simulink model "buck_converter_closed_loop_with_cascaded_comp"  (R2019a)
settings: Solver=VariableStepAuto  StartTime=0.0  StopTime=0.5  MaxStep=1e-6  RelTol=1e-6
values from neighbouring files (symbols this model uses):
  C = 68e-6    (= 6.8e-05)    [parameters_closed_loop_with_various_load.m]
  Cc2 = 2.8e-9    (= 2.8e-09)    [parameters_closed_loop_with_various_load.m]
  Cc3 = 470e-12    (= 4.7e-10)    [parameters_closed_loop_with_various_load.m]
  Cv2 = 0.94e-6    (= 9.4e-07)    [parameters_closed_loop_with_various_load.m]
  Cv3 = 0.056e-6    (= 5.6e-08)    [parameters_closed_loop_with_various_load.m]
  H = 0.5    [parameters_closed_loop_with_various_load.m]
  L = 68e-6    (= 6.8e-05)    [parameters_closed_loop_with_various_load.m]
  R = V/I    (= 0.363636363636)    [parameters_closed_loop_with_various_load.m]
  Ra = 2e3    (= 2000)    [parameters_closed_loop_with_various_load.m]
  Rb = 2e3    (= 2000)    [parameters_closed_loop_with_various_load.m]
  Rc1 = 1e3    (= 1000)    [parameters_closed_loop_with_various_load.m]
  Rc2 = 13.3404e3    (= 13340.4)    [parameters_closed_loop_with_various_load.m]
  Resr = 9e-3    (= 0.009)    [parameters_closed_loop_with_various_load.m]
  Rf = 0.3    [parameters_closed_loop_with_various_load.m]
  RL = 30e-3    (= 0.03)    [parameters_closed_loop_with_various_load.m]
  Rv2 = 546    [parameters_closed_loop_with_various_load.m]
  V = 1.2    [parameters_closed_loop_with_various_load.m]
  Vm = 5    [parameters_closed_loop_with_various_load.m]
undefined symbols (not defined in the file or in its folder): Rcomp_1
libraries: powerlib x64, simulink x1, powerlib_meascontrol x1
settings Model: Creator=Görkem  LastModifiedBy=Görkem
settings SolverCC: ZeroCrossAlgorithm=Adaptive
settings DebuggingCC: IgnoredZcDiagnostic=none

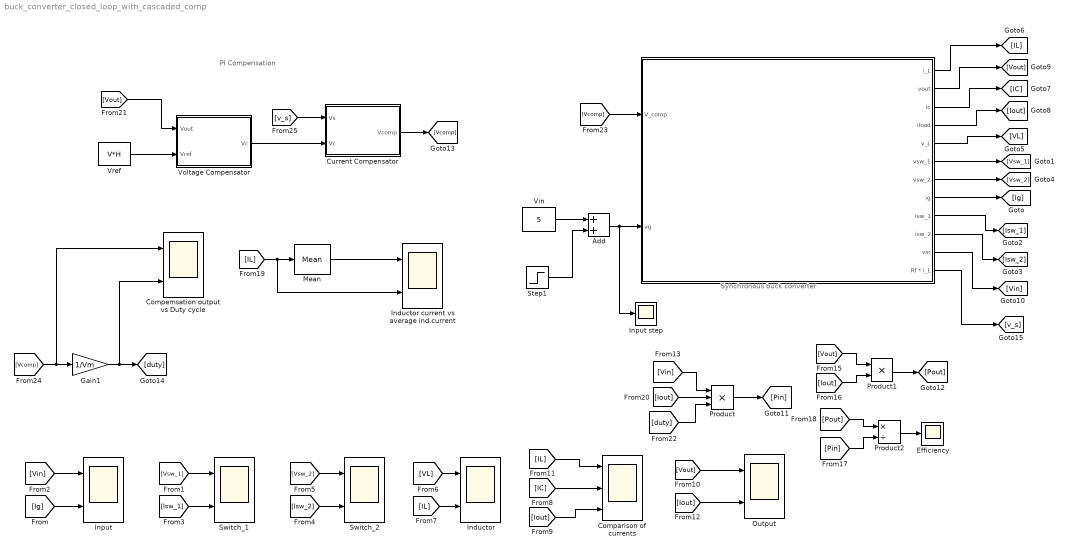
== system buck_converter_closed_loop_with_cascaded_comp ==
  note: PI Compensation
  note: Synchronous buck converter
  "   " : Subsystem
  Add : Sum
  Comparison of currents : Scope  NumInputPorts=3
  Compemsation output vs Duty cycle : Scope  NumInputPorts=2
  Current Compensator : Subsystem
  Efficiency : Scope
  Gain1 : Gain  Gain=1/Vm
  Inductor : Scope  NumInputPorts=2
  Inductor current vs average ind.current : Scope  NumInputPorts=2
  Input : Scope  NumInputPorts=2
  Input step : Scope
  Mean : powerlib_meascontrol/Measurements/Mean  Freq=fsw  Vinit=0  Ts=0
      settings: SourceProductName=Simscape Electrical
  "Output " : Scope  NumInputPorts=2
  Product : Product  Inputs=3
  Product1 : Product
  Product2 : Product  Inputs=*/
  Step1 : Step  Time=0.15  SampleTime=0
  Switch_1 : Scope  NumInputPorts=2
  Switch_2 : Scope  NumInputPorts=2
  Vin : Constant  Value=5
  "Voltage Compensator " : Subsystem
  Vref : Constant  Value=V*H
  wires:
  [Vsw_1] -> Switch_1/1
  [Isw_1] -> Switch_1/2
  [Vsw_2] -> Switch_2/1
  [Isw_2] -> Switch_2/2
  [VL] -> Inductor/1
  [IL] -> Inductor/2
  [IL] -> Comparison of currents/1
  [IC] -> Comparison of currents/2
  [Iout] -> Comparison of currents/3
  [Vout] -> "Output "/1
  [Iout] -> "Output "/2
  [Vin] -> Input/1
  [Ig] -> Input/2
  [Vin] -> Product/1
  [Iout] -> Product/2
  [Vout] -> Product1/1
  [Iout] -> Product1/2
  Product1/1 -> [Pout]
  Product/1 -> [Pin]
  [Pout] -> Product2/1
  [Pin] -> Product2/2
  Product2/1 -> Efficiency/1
  [duty] -> Product/3
  "   "/4(iload) -> [Iout]
  "   "/3(ic) -> [IC]
  "   "/2(vout) -> [Vout]
  "   "/1(i_L) -> [IL]
  "   "/5(v_L) -> [VL]
  "   "/6(vsw_1) -> [Vsw_1]
  "   "/7(vsw_2) -> [Vsw_2]
  "   "/8(ig) -> [Ig]
  "   "/9(isw_1) -> [Isw_1]
  "   "/10(isw_2) -> [Isw_2]
  "   "/11(vin) -> [Vin]
  [IL] -> Inductor current vs average ind.current/2, Mean/1
  Mean/1 -> Inductor current vs average ind.current/1
  [Vout] -> "Voltage Compensator "/1(Vout)
  [Vcomp] -> "   "/1(V_comp)
  [Vcomp] -> Compemsation output vs Duty cycle/1, Gain1/1
  Gain1/1 -> Compemsation output vs Duty cycle/2, [duty]
  "Voltage Compensator "/1(Vc) -> Current Compensator/2(Vc)
  "   "/12(Rf * i_L) -> [v_s]
  [v_s] -> Current Compensator/1(Vs)
  Vin/1 -> Add/1
  Add/1 -> Input step/1, "   "/2(vg)
  Vref/1 -> "Voltage Compensator "/2(Vref)
  Step1/1 -> Add/2
  Current Compensator/1(Vcomp) -> [Vcomp]

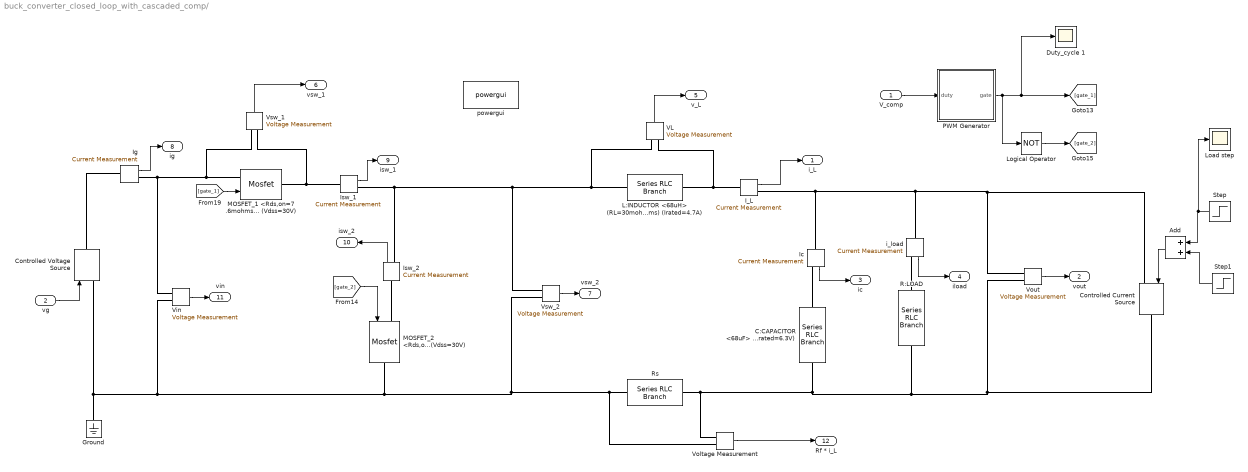
== system buck_converter_closed_loop_with_cascaded_comp/    ==
  V_comp : Inport
  vg : Inport  Port=2
  Add : Sum
  C:CAPACITOR <68uF> (Resr=9mohms) (Vrated=6.3V) : powerlib/Elements/Series RLC Branch  LConnTagsString=__new0  RConnTagsString=__new0  BranchType=RC  Resistance=Resr  Inductance=1e-3  SetiL0=off  InitialCurrent=0  Capacitance=C  Setx0=off  InitialVoltage=0  Measurements=None
      settings: SourceProductName=Simscape Electrical
  Controlled Current Source : powerlib/Electrical Sources/Controlled Current Source  Initialize=on  Source_Type=AC  Amplitude=0  Phase=0  Frequency=0  Measurements=None
      settings: SourceProductName=Simscape Electrical
  Controlled Voltage Source : powerlib/Electrical Sources/Controlled Voltage Source  Initialize=on  Source_Type=DC  Amplitude=0  Phase=0  Frequency=0  Measurements=None
      settings: SourceProductName=Simscape Electrical
  Duty_cycle 1 : Scope
  Ground : powerlib/Elements/Ground  LConnTagsString=a
      settings: SourceProductName=Simscape Electrical
  I_L : powerlib/Measurements/Current Measurement  PhasorSimulation=off  OutputType=Complex  PSBequivalent=0
      settings: SourceProductName=Simscape Electrical
  Ic : powerlib/Measurements/Current Measurement  PhasorSimulation=off  OutputType=Complex  PSBequivalent=0
      settings: SourceProductName=Simscape Electrical
  Ig : powerlib/Measurements/Current Measurement  PhasorSimulation=off  OutputType=Complex  PSBequivalent=0
      settings: SourceProductName=Simscape Electrical
  Isw_1 : powerlib/Measurements/Current Measurement  PhasorSimulation=off  OutputType=Complex  PSBequivalent=0
      settings: SourceProductName=Simscape Electrical
  Isw_2 : powerlib/Measurements/Current Measurement  PhasorSimulation=off  OutputType=Complex  PSBequivalent=0
      settings: SourceProductName=Simscape Electrical
  "L:INDUCTOR <68uH> (RL=30mohms) (Irated=4.7A) " : powerlib/Elements/Series RLC Branch  LConnTagsString=__new0  RConnTagsString=__new0  BranchType=RL  Resistance=RL  Inductance=L  SetiL0=off  InitialCurrent=0  Capacitance=1e-6  Setx0=off  InitialVoltage=0  Measurements=None
      settings: SourceProductName=Simscape Electrical
  Load step : Scope
  Logical Operator : Logic  Operator=NOT  AllPortsSameDT=off  OutDataTypeStr=boolean
  MOSFET_1 <Rds,on=7.6mohms> (Ids=7A) (Vdss=30V) : powerlib/Power Electronics/Mosfet  Ron=Rdson  Lon=0  Rd=0  Vfd=Vf  IC=0  Rs=1e5  Cs=inf  Measurements=off
      settings: SourceProductName=Simscape Electrical
  MOSFET_2 <Rds,on=7.6mohms> (Ids=7A) (Vdss=30V) : powerlib/Power Electronics/Mosfet  Ron=Rdson  Lon=0  Rd=0  Vfd=Vf  IC=0  Rs=1e5  Cs=inf  Measurements=off
      settings: SourceProductName=Simscape Electrical
  PWM Generator : Subsystem
  "R:LOAD " : powerlib/Elements/Series RLC Branch  LConnTagsString=__new0  RConnTagsString=__new0  BranchType=R  Resistance=R  Inductance=1e-3  SetiL0=off  InitialCurrent=0  Capacitance=47e-6  Setx0=off  InitialVoltage=0  Measurements=None
      settings: SourceProductName=Simscape Electrical
  Rs : powerlib/Elements/Series RLC Branch  LConnTagsString=__new0  RConnTagsString=__new0  BranchType=R  Resistance=Rf  Inductance=1e-3  SetiL0=off  InitialCurrent=0  Capacitance=47e-6  Setx0=off  InitialVoltage=0  Measurements=None
      settings: SourceProductName=Simscape Electrical
  Step : Step  Time=0.05  SampleTime=0
  Step1 : Step  Time=0.1  After=-1  SampleTime=0
  VL : powerlib/Measurements/Voltage Measurement  PhasorSimulation=off  OutputType=Complex  PSBequivalent=0
      settings: SourceProductName=Simscape Electrical
  Vin : powerlib/Measurements/Voltage Measurement  PhasorSimulation=off  OutputType=Complex  PSBequivalent=0
      settings: SourceProductName=Simscape Electrical
  Voltage Measurement : powerlib/Measurements/Voltage Measurement  PhasorSimulation=off  OutputType=Complex  PSBequivalent=0
  Vout : powerlib/Measurements/Voltage Measurement  PhasorSimulation=off  OutputType=Complex  PSBequivalent=0
      settings: SourceProductName=Simscape Electrical
  Vsw_1 : powerlib/Measurements/Voltage Measurement  PhasorSimulation=off  OutputType=Complex  PSBequivalent=0
      settings: SourceProductName=Simscape Electrical
  Vsw_2 : powerlib/Measurements/Voltage Measurement  PhasorSimulation=off  OutputType=Complex  PSBequivalent=0
      settings: SourceProductName=Simscape Electrical
  i_load : powerlib/Measurements/Current Measurement  PhasorSimulation=off  OutputType=Complex  PSBequivalent=0
      settings: SourceProductName=Simscape Electrical
  powergui : powerlib/powergui  Priority=1  SimulationMode=Continuous  SampleTime=50e-6  frequency=60  Iterations=50  frequencyindice=0  Pbase=100e6  ErrMax=1e-4  UnitsV=kV  UnitsW=MW  buscounter=0  FunctionMessages=off  echomessages=off  EnableUseOfTLC=off  CurrentSourceSwitches=off  DisableSnubberDevices=off  DisableRonSwitches=off  DisableVfSwitches=off  DisplayEquations=off  AutomaticDiscreteSolvers=off  SolverType=Tustin/Backward Euler (TBE)  Interpol=off  ExternalGateDelay=off  methode=off  Ts=100  x0status=blocks  SPID=on  SwTol=0  HookPort=off  NonlinearTolerance=0  nMaxIteration=15  ContinueOnMaxIteration=off  RestoreLinks=warning  ResistiveCurrentMeasurement=off  Frange=[0:2:500]  Ylog=off  Xlog=on  ShowGrid=off  save=off  variable=ZData  structure=0  ZoomFFT=off  StartTime=0.0  cycles=1  DisplayStyle=1  fundamental=60  FreqAxis=off  MaxFrequency=1000  frequencyindicesteady=1  RmsSteady=1  display=off
      settings: SourceProductName=Simscape Electrical
  i_L : Outport
  vout : Outport  Port=2
  ic : Outport  Port=3
  iload : Outport  Port=4
  v_L : Outport  Port=5
  vsw_1 : Outport  Port=6
  vsw_2 : Outport  Port=7
  ig : Outport  Port=8
  isw_1 : Outport  Port=9
  isw_2 : Outport  Port=10
  vin : Outport  Port=11
  Rf * i_L : Outport  Port=12
  wires:
  Logical Operator/1 -> [gate_2]
  V_comp/1 -> PWM Generator/1(duty)
  [gate_2] -> MOSFET_2 <Rds,on=7.6mohms> (Ids=7A) (Vdss=30V)/1
  i_load/1 -> iload/1
  Vout/1 -> vout/1
  I_L/1 -> i_L/1
  Ic/1 -> ic/1
  Vsw_2/1 -> vsw_2/1
  [gate_1] -> MOSFET_1 <Rds,on=7.6mohms> (Ids=7A) (Vdss=30V)/1
  PWM Generator/1(gate) -> Logical Operator/1, Duty_cycle 1/1, [gate_1]
  Ig/1 -> ig/1
  Isw_1/1 -> isw_1/1
  VL/1 -> v_L/1
  Isw_2/1 -> isw_2/1
  Vin/1 -> vin/1
  Vsw_1/1 -> vsw_1/1
  vg/1 -> Controlled Voltage Source/1
  Voltage Measurement/1 -> Rf * i_L/1
  Step/1 -> Load step/1, Add/1
  Step1/1 -> Add/2
  Add/1 -> Controlled Current Source/1
  connections:
  MOSFET_1 <Rds,on=7.6mohms> (Ids=7A) (Vdss=30V)/LConn1 -- Vin/LConn1 -- Ig/RConn1 -- Vsw_1/LConn1
  Controlled Voltage Source/LConn1 -- Ground/LConn1 -- Vin/LConn2 -- Voltage Measurement/LConn2 -- Rs/RConn1 -- Vsw_2/LConn2 -- MOSFET_2 <Rds,on=7.6mohms> (Ids=7A) (Vdss=30V)/RConn1
  Isw_1/RConn1 -- Isw_2/RConn1 -- Vsw_2/LConn1 -- "L:INDUCTOR <68uH> (RL=30mohms) (Irated=4.7A) "/LConn1 -- VL/LConn1
  I_L/RConn1 -- i_load/LConn1 -- Controlled Current Source/LConn1 -- Vout/LConn1 -- Ic/LConn1
  Controlled Voltage Source/RConn1 -- Ig/LConn1
  I_L/LConn1 -- VL/LConn2 -- "L:INDUCTOR <68uH> (RL=30mohms) (Irated=4.7A) "/RConn1
  Vsw_1/LConn2 -- Isw_1/LConn1 -- MOSFET_1 <Rds,on=7.6mohms> (Ids=7A) (Vdss=30V)/RConn1
  MOSFET_2 <Rds,on=7.6mohms> (Ids=7A) (Vdss=30V)/LConn1 -- Isw_2/LConn1
  Ic/RConn1 -- C:CAPACITOR <68uF> (Resr=9mohms) (Vrated=6.3V)/LConn1
  i_load/RConn1 -- "R:LOAD "/LConn1
  "R:LOAD "/RConn1 -- C:CAPACITOR <68uF> (Resr=9mohms) (Vrated=6.3V)/RConn1 -- Voltage Measurement/LConn1 -- Rs/LConn1 -- Controlled Current Source/RConn1 -- Vout/LConn2

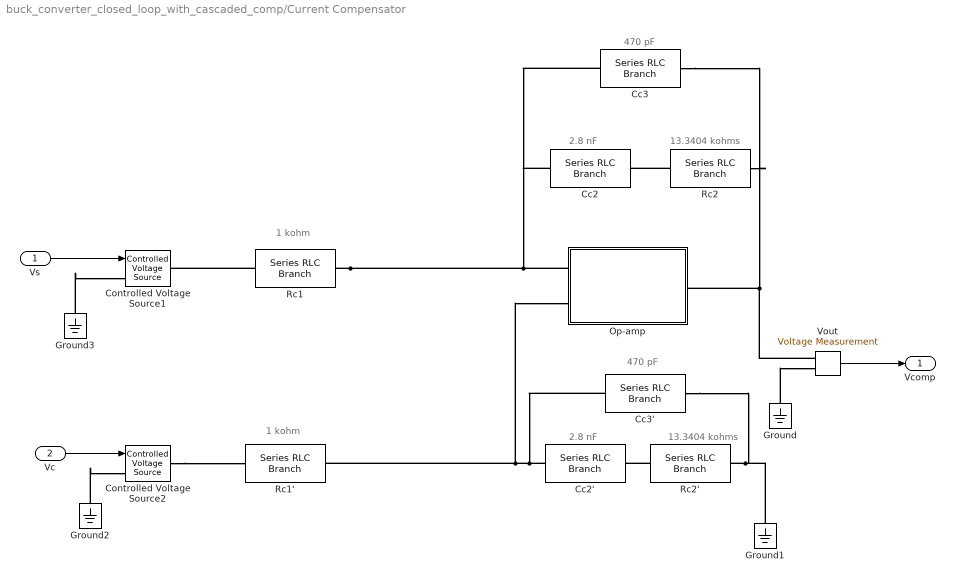
== system buck_converter_closed_loop_with_cascaded_comp/Current Compensator ==
  note: 1 kohm
  note: 13.3404 kohms
  note: 2.8 nF
  note: 1 kohm
  note: 2.8 nF
  note: 13.3404 kohms
  note: 470 pF
  note: 470 pF
  Vs : Inport
  Vc : Inport  Port=2
  "Cc2 " : powerlib/Elements/Series RLC Branch  LConnTagsString=__new0  RConnTagsString=__new0  BranchType=C  Resistance=Rcomp_1*0.98  Inductance=1e-3  SetiL0=off  InitialCurrent=0  Capacitance=Cc2  Setx0=off  InitialVoltage=0  Measurements=None
  "Cc2' " : powerlib/Elements/Series RLC Branch  LConnTagsString=__new0  RConnTagsString=__new0  BranchType=C  Resistance=Rcomp_1*0.98  Inductance=1e-3  SetiL0=off  InitialCurrent=0  Capacitance=Cc2  Setx0=off  InitialVoltage=0  Measurements=None
  Cc3 : powerlib/Elements/Series RLC Branch  LConnTagsString=__new0  RConnTagsString=__new0  BranchType=C  Resistance=Rcomp_1*0.98  Inductance=1e-3  SetiL0=off  InitialCurrent=0  Capacitance=Cc3  Setx0=off  InitialVoltage=0  Measurements=None
  Cc3' : powerlib/Elements/Series RLC Branch  LConnTagsString=__new0  RConnTagsString=__new0  BranchType=C  Resistance=Rcomp_1*0.98  Inductance=1e-3  SetiL0=off  InitialCurrent=0  Capacitance=Cc3  Setx0=off  InitialVoltage=0  Measurements=None
  Controlled Voltage Source1 : powerlib/Electrical Sources/Controlled Voltage Source  Initialize=on  Source_Type=AC  Amplitude=0  Phase=0  Frequency=0  Measurements=None
  Controlled Voltage Source2 : powerlib/Electrical Sources/Controlled Voltage Source  Initialize=on  Source_Type=AC  Amplitude=0  Phase=0  Frequency=0  Measurements=None
  Ground{,1..3} (4 alike) : powerlib/Elements/Ground  LConnTagsString=a
  Op-amp : Subsystem
      mask Display: image('C:\Users\Görkem\Desktop\Ekran Alıntısı.PNG');
  Rc1 : powerlib/Elements/Series RLC Branch  LConnTagsString=__new0  RConnTagsString=__new0  BranchType=R  Resistance=Rc1  Inductance=1e-3  SetiL0=off  InitialCurrent=0  Capacitance=1e-6  Setx0=off  InitialVoltage=0  Measurements=None
  Rc1' : powerlib/Elements/Series RLC Branch  LConnTagsString=__new0  RConnTagsString=__new0  BranchType=R  Resistance=Rc1  Inductance=1e-3  SetiL0=off  InitialCurrent=0  Capacitance=1e-6  Setx0=off  InitialVoltage=0  Measurements=None
  Rc2 : powerlib/Elements/Series RLC Branch  LConnTagsString=__new0  RConnTagsString=__new0  BranchType=R  Resistance=Rc2  Inductance=1e-3  SetiL0=off  InitialCurrent=0  Capacitance=56e-6  Setx0=off  InitialVoltage=0  Measurements=None
  Rc2' : powerlib/Elements/Series RLC Branch  LConnTagsString=__new0  RConnTagsString=__new0  BranchType=R  Resistance=Rc2  Inductance=1e-3  SetiL0=off  InitialCurrent=0  Capacitance=56e-6  Setx0=off  InitialVoltage=0  Measurements=None
  Vout : powerlib/Measurements/Voltage Measurement  PhasorSimulation=off  OutputType=Complex  PSBequivalent=0
  Vcomp : Outport
  wires:
  Vout/1 -> Vcomp/1
  Vs/1 -> Controlled Voltage Source1/1
  Vc/1 -> Controlled Voltage Source2/1
  connections:
  Vout/LConn1 -- Op-amp/RConn1 -- Rc2/RConn1 -- Cc3/RConn1
  Rc2/LConn1 -- "Cc2 "/RConn1
  Rc2'/LConn1 -- "Cc2' "/RConn1
  Ground/LConn1 -- Vout/LConn2
  Rc2'/RConn1 -- Ground1/LConn1 -- Cc3'/RConn1
  Ground3/LConn1 -- Controlled Voltage Source1/LConn1
  Ground2/LConn1 -- Controlled Voltage Source2/LConn1
  Rc1/RConn1 -- Op-amp/LConn1 -- Cc3/LConn1 -- "Cc2 "/LConn1
  Controlled Voltage Source2/RConn1 -- Rc1'/LConn1
  Cc3'/LConn1 -- "Cc2' "/LConn1 -- Op-amp/LConn2 -- Rc1'/RConn1
  Rc1/LConn1 -- Controlled Voltage Source1/RConn1

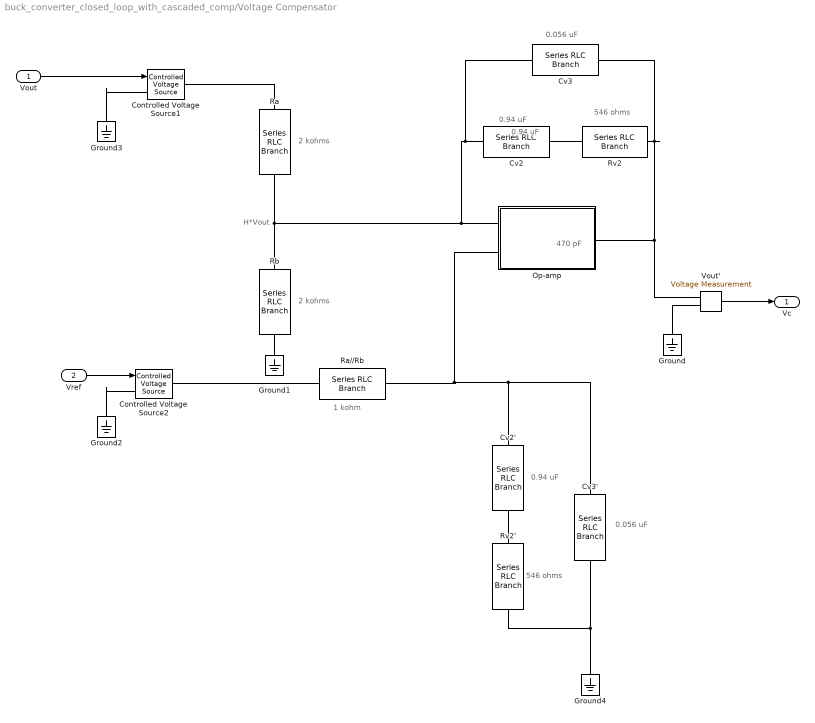
== system buck_converter_closed_loop_with_cascaded_comp/Voltage Compensator  ==
  note: H*Vout
  note: 546 ohms
  note: 0.94 uF
  note: 0.056 uF
  note: 0.94 uF
  note: 0.94 uF
  note: 546 ohms
  note: 0.056 uF
  note: 2 kohms
  note: 2 kohms
  note: 1 kohm
  note: 470 pF
  Vout : Inport
  Vref : Inport  Port=2
  Controlled Voltage Source1 : powerlib/Electrical Sources/Controlled Voltage Source  Initialize=on  Source_Type=AC  Amplitude=0  Phase=0  Frequency=0  Measurements=None
  Controlled Voltage Source2 : powerlib/Electrical Sources/Controlled Voltage Source  Initialize=on  Source_Type=AC  Amplitude=0  Phase=0  Frequency=0  Measurements=None
  "Cv2 " : powerlib/Elements/Series RLC Branch  LConnTagsString=__new0  RConnTagsString=__new0  BranchType=C  Resistance=Rcomp_1*0.98  Inductance=1e-3  SetiL0=off  InitialCurrent=0  Capacitance=Cv2  Setx0=off  InitialVoltage=0  Measurements=None
  Cv2' : powerlib/Elements/Series RLC Branch  LConnTagsString=__new0  RConnTagsString=__new0  BranchType=C  Resistance=Rcomp_1*0.98  Inductance=1e-3  SetiL0=off  InitialCurrent=0  Capacitance=Cv2  Setx0=off  InitialVoltage=0  Measurements=None
  Cv3 : powerlib/Elements/Series RLC Branch  LConnTagsString=__new0  RConnTagsString=__new0  BranchType=C  Resistance=Rcomp_1*0.98  Inductance=1e-3  SetiL0=off  InitialCurrent=0  Capacitance=Cv3  Setx0=off  InitialVoltage=0  Measurements=None
  Cv3' : powerlib/Elements/Series RLC Branch  LConnTagsString=__new0  RConnTagsString=__new0  BranchType=C  Resistance=Rcomp_1*0.98  Inductance=1e-3  SetiL0=off  InitialCurrent=0  Capacitance=Cv3  Setx0=off  InitialVoltage=0  Measurements=None
  Ground{,1..4} (5 alike) : powerlib/Elements/Ground  LConnTagsString=a
  Op-amp : Subsystem
      mask Display: image('C:\Users\Görkem\Desktop\Ekran Alıntısı.PNG');
  Ra : powerlib/Elements/Series RLC Branch  LConnTagsString=__new0  RConnTagsString=__new0  BranchType=R  Resistance=Ra  Inductance=1e-3  SetiL0=off  InitialCurrent=0  Capacitance=1e-6  Setx0=off  InitialVoltage=0  Measurements=None
  Ra//Rb : powerlib/Elements/Series RLC Branch  LConnTagsString=__new0  RConnTagsString=__new0  BranchType=R  Resistance=1e3  Inductance=1e-3  SetiL0=off  InitialCurrent=0  Capacitance=56e-6  Setx0=off  InitialVoltage=0  Measurements=None
  Rb : powerlib/Elements/Series RLC Branch  LConnTagsString=__new0  RConnTagsString=__new0  BranchType=R  Resistance=Rb  Inductance=1e-3  SetiL0=off  InitialCurrent=0  Capacitance=1e-6  Setx0=off  InitialVoltage=0  Measurements=None
  Rv2 : powerlib/Elements/Series RLC Branch  LConnTagsString=__new0  RConnTagsString=__new0  BranchType=R  Resistance=Rv2  Inductance=1e-3  SetiL0=off  InitialCurrent=0  Capacitance=56e-6  Setx0=off  InitialVoltage=0  Measurements=None
  Rv2' : powerlib/Elements/Series RLC Branch  LConnTagsString=__new0  RConnTagsString=__new0  BranchType=R  Resistance=Rv2  Inductance=1e-3  SetiL0=off  InitialCurrent=0  Capacitance=56e-6  Setx0=off  InitialVoltage=0  Measurements=None
  Vout' : powerlib/Measurements/Voltage Measurement  PhasorSimulation=off  OutputType=Complex  PSBequivalent=0
  Vc : Outport
  wires:
  Vout'/1 -> Vc/1
  Vout/1 -> Controlled Voltage Source1/1
  Vref/1 -> Controlled Voltage Source2/1
  connections:
  Vout'/LConn1 -- Cv3/RConn1 -- Rv2/RConn1 -- Op-amp/RConn1
  Rv2/LConn1 -- "Cv2 "/RConn1
  Ground/LConn1 -- Vout'/LConn2
  Ground3/LConn1 -- Controlled Voltage Source1/LConn1
  Ground2/LConn1 -- Controlled Voltage Source2/LConn1
  Op-amp/LConn2 -- Ra//Rb/LConn1 -- Cv3'/LConn1 -- Cv2'/LConn1
  Controlled Voltage Source1/RConn1 -- Ra/LConn1
  Op-amp/LConn1 -- Ra/RConn1 -- Rb/LConn1 -- "Cv2 "/LConn1 -- Cv3/LConn1
  Ground1/LConn1 -- Rb/RConn1
  Cv2'/RConn1 -- Rv2'/LConn1
  Rv2'/RConn1 -- Ground4/LConn1 -- Cv3'/RConn1
  Controlled Voltage Source2/RConn1 -- Ra//Rb/RConn1

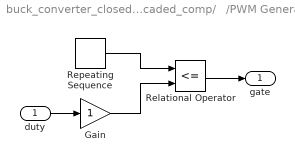
== system buck_converter_closed_loop_with_cascaded_comp/   /PWM Generator ==
  duty : Inport
  Gain : Gain
  Relational Operator : RelationalOperator  Operator=<=  OutDataTypeStr=boolean  RndMeth=Simplest
  Repeating Sequence : simulink/Sources/Repeating Sequence  rep_seq_t=[0 0.5/50000 1/50000]  rep_seq_y=[0 Vm 0]
  gate : Outport
  wires:
  Repeating Sequence/1 -> Relational Operator/1
  Relational Operator/1 -> gate/1
  duty/1 -> Gain/1
  Gain/1 -> Relational Operator/2

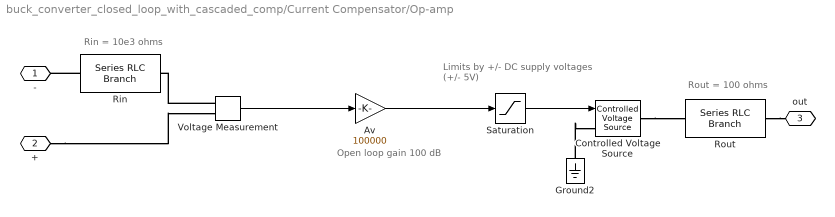
== system buck_converter_closed_loop_with_cascaded_comp/Current Compensator/Op-amp ==
  note: Open loop gain
      | 	100 dB
  note: Limits by +/- DC supply voltages
      |                   (+/- 5V)
  note: Rin = 10e3 ohms
  note: Rout = 100 ohms
  Av : Gain  Gain=100000
  Controlled Voltage Source : powerlib/Electrical Sources/Controlled Voltage Source  Initialize=on  Source_Type=AC  Amplitude=0  Phase=0  Frequency=0  Measurements=None
  Ground2 : powerlib/Elements/Ground  LConnTagsString=a
  Rin : powerlib/Elements/Series RLC Branch  LConnTagsString=__new0  RConnTagsString=__new0  BranchType=R  Resistance=10e3  Inductance=1e-3  SetiL0=off  InitialCurrent=0  Capacitance=1e-6  Setx0=off  InitialVoltage=0  Measurements=None
  Rout : powerlib/Elements/Series RLC Branch  LConnTagsString=__new0  RConnTagsString=__new0  BranchType=R  Resistance=100  Inductance=1e-3  SetiL0=off  InitialCurrent=0  Capacitance=1e-6  Setx0=off  InitialVoltage=0  Measurements=None
  Saturation : Saturate  UpperLimit=5  LowerLimit=-5
  Voltage Measurement : powerlib/Measurements/Voltage Measurement  PhasorSimulation=off  OutputType=Complex  PSBequivalent=0
  - : PMIOPort  Side=Left
  + : PMIOPort  Port=2  Side=Left
  out : PMIOPort  Port=3  Side=Right
  wires:
  Av/1 -> Saturation/1
  Voltage Measurement/1 -> Av/1
  Saturation/1 -> Controlled Voltage Source/1
  connections:
  Controlled Voltage Source/RConn1 -- Rout/LConn1
  Ground2/LConn1 -- Controlled Voltage Source/LConn1
  Voltage Measurement/LConn2 -- Rin/RConn1
  +/RConn1 -- Voltage Measurement/LConn1
  Rin/LConn1 -- -/RConn1
  Rout/RConn1 -- out/RConn1

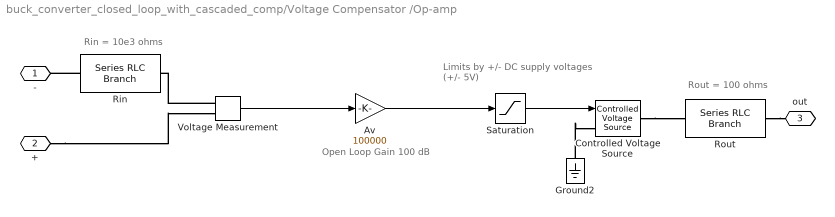
== system buck_converter_closed_loop_with_cascaded_comp/Voltage Compensator /Op-amp ==
  note: Open Loop Gain
      | 	  100 dB
  note: Limits by +/- DC supply voltages
      |                   (+/- 5V)
  note: Rin = 10e3 ohms
  note: Rout = 100 ohms
  Av : Gain  Gain=100000
  Controlled Voltage Source : powerlib/Electrical Sources/Controlled Voltage Source  Initialize=on  Source_Type=AC  Amplitude=0  Phase=0  Frequency=0  Measurements=None
  Ground2 : powerlib/Elements/Ground  LConnTagsString=a
  Rin : powerlib/Elements/Series RLC Branch  LConnTagsString=__new0  RConnTagsString=__new0  BranchType=R  Resistance=10e3  Inductance=1e-3  SetiL0=off  InitialCurrent=0  Capacitance=1e-6  Setx0=off  InitialVoltage=0  Measurements=None
  Rout : powerlib/Elements/Series RLC Branch  LConnTagsString=__new0  RConnTagsString=__new0  BranchType=R  Resistance=100  Inductance=1e-3  SetiL0=off  InitialCurrent=0  Capacitance=1e-6  Setx0=off  InitialVoltage=0  Measurements=None
  Saturation : Saturate  UpperLimit=5  LowerLimit=-5
  Voltage Measurement : powerlib/Measurements/Voltage Measurement  PhasorSimulation=off  OutputType=Complex  PSBequivalent=0
  - : PMIOPort  Side=Left
  + : PMIOPort  Port=2  Side=Left
  out : PMIOPort  Port=3  Side=Right
  wires:
  Av/1 -> Saturation/1
  Voltage Measurement/1 -> Av/1
  Saturation/1 -> Controlled Voltage Source/1
  connections:
  Controlled Voltage Source/RConn1 -- Rout/LConn1
  Ground2/LConn1 -- Controlled Voltage Source/LConn1
  Voltage Measurement/LConn2 -- Rin/RConn1
  +/RConn1 -- Voltage Measurement/LConn1
  Rin/LConn1 -- -/RConn1
  Rout/RConn1 -- out/RConn1
